simulink model "CAVE_MachE_Simulink_250904"  (R2024a)
settings: configuration reference "ConfigSetDesktopFixedStep" (kept outside this file)
PreLoadFcn:
  | VSS_BICYCLE=Simulink.Variant('Dual=0');
  | VSS_DUAL=Simulink.Variant('Dual=1');
  | Dual=1;
  | load('DriveCycle2.mat')
PostLoadFcn:
  | if any(exist('dsrtsu_mdlpostloadfcn', 'file') ~= 0), dsrtsu_mdlpostloadfcn('Execute', bdroot); end
InitFcn:
  | , if any(exist('rtifpga_mdlclblib', 'file') ~= 0), rtifpga_mdlclblib('Init', bdroot); end,
  | , if any(exist('dsmpb_private', 'file') ~= 0), dsmpb_private('dsmpb_mdlclblib', 'Init', bdroot); end,
  | load('DriveCycle2.mat')
model workspace (MAT data in the model file):
  Gas = 0.383333333333
undefined symbols (not defined in the file or in its folder): AccelCmd, ActTqLF_Nm_, ActTqLR_Nm_, ActTqRF_Nm_, ActTqRR_Nm_, BattChargeLimitMaxPwr, BattChargeLimitSocBpts, BattChargeLimitTbl, BattChrgCapcty, BattDischargeLimitSocBpts, BattDischargeLimitTbl, BattDischargeMaxPwr, BattNumCellsParallel, BattNumCellsSeries, BattOpenVoltCapBpts, BattOpenVoltTbl, BattResistSocBpts, BattResistTbl, BattResistTempBpts, BrakeMaxPrs, BrakeMaxTrq, ChassisDistCg2FrontAxle, ChassisDistCg2RearAxle, ChassisVehMass, CltchCmd, CoastDown, DecelCmd, DiffRatio, DiscIntNeverNeededParam, EnvGravCnst, EnvPrs, EnvTemp, FuelSpecificGrav, GearCmd, h, InitStates, lgSw, limitedMCT, MCT, MtrEffSpdBpts, MtrEffTbl, MtrEffTrqBpts, MtrPwrMax, MtrTrqMax, pMCT, RealSimPara, Ref_speed, Ref_time, SteeringCmd, SupvsryCtrlRegenBrkCutOffTbl, SupvsryCtrlRegenSpdBpts, TestScnrioCycleNum, US06, VEH
libraries: VSIGenLib x179, simulink x166, etargetslib x112, dsmpblib x58, vehdynlibtire x36, autolibshared x29, vehdynlibsuspension x21, vehdynlibtirecommon x21, autolibutils x15, CarMaker4SL x12, VsrLibWheel x12, autolibpowerinfoutils x9
(part 1 of 43)
PreSaveFcn:
  | , if any(exist('dsmpb_private', 'file') ~= 0), dsmpb_private('dsmpb_mdlclblib', 'PreSave', bdroot); end,
CloseFcn:
  | , if any(exist('dsmpb_private', 'file') ~= 0), dsmpb_private('dsmpb_mdlclblib', 'Close', bdroot); end,
settings Model: DataDictionary=DdPassengerEv.sldd  DSMPB_ID_DATA={'18088',struct('BlockId','f88c42c2-e70e-4436-bd85-ff34452e836e','SignalIds',{{'1df572a0-f117-4729-9091-2c1a0a26ec90','0824b86c-995c-4624-95de-4f5a118cf0f7','1af539eb-325a-4e38-9107-84d6b0267392','ebb0fa34-559f-4fe0-b409-8a817ae8753c','d7145080-d35d-4c02-8c9e-cf76ffb14dc2','5075bfde-4142-4aeb-b309-025b37120541','abbab0bd-1456-4252-a37b-ee5f55ea0579','b5d617b8-bb24-4539-9145-e591a0a295f8','7df03788-1936-4801-98c0-dd7f6dfcacba','19949bfb-f246-4995-90e8-29a3751a0fa7','9454b59a-aedd-4270-89a6-1cca43305823','37cf720c-23c2-4b6d-8589-7b035c806643','98db9f76-eafd-4d54-90d2-d997d73b87d4','ff589fc8-5b21-4798-a75e-d26fc35c1fa1','e61b2882-e27e-4f06-b730-5e5281621b34','6605e0e6-8bf3-4a45-a0b0-4b9c1cf463f3','0d0f5161-daad-47a1-bb1d-ec2adbc183ca','48ba6675-0966-4a1c-b127-4f76dca3de94','3c897f11-b2eb-4eb8-b88f-7b7e913c6e41','378f468e-364f-43c5-91f9-fc8ddef6aca6','9c7f20ac-956d-4c19-bdea-31a2a3930ea2','bc252920-9c7c-4b91-a017-ee1d69e3f03c','a5e7a104-8664-4690-a58a-7cbf05737866','fe1cfa34-9b23-4225-85e3-0403f07d36e7','ab40d80a-815e-4994-aacd-e42d283f5b3a','2a4143b2-c438-4d42-997d-0587141eb8f0','2686c37a-8724-40b3-99fb-f8873ba286b8','3707aa1b-88c1-4f14-8f25-f346aa75c252','7413af4b-f834-4020-ad34-3dd98c546e0c','3445835b-9a90-4408-a32d-d76b66b0385b','23c9a144-1259-4fa3-9a16-4a32a7eadff9','5b4206b0-ea89-4111-86f7-7a4fd8c76b72','85c84ea6-72b6-4ccb-9199-727b305580c3','97bb0073-9d03-44a9-972d-49a0eb465678','8c3f0698-b0b6-4624-aa00-3a3096f7cc2f','c968922f-253e-433f-ad46-daf21e902962','21ad150a-19dc-415b-bc1b-b39528ec9221','a3572415-9467-4ff8-a492-c6c1b3cb1b64','700ac678-fb53-40b6-8e97-9eeffe7a1ca8','14ed5f8b-aa1d-402b-b493-5622a729893d','bdbcc0b3-c6a4-485e-8fbf-8c12a8df89e7','7a19cc2b-f06b-466f-ae52-fb8ac6fb0258','87deda6a-2251-4462-8ae0-a20845c776d4','41874d9b-304a-4265-a3a1-69d5c58383ea'}}),'18719',struct('BlockId','79daabbd-4df4-4017-ba65-d977f7e6cd2f','SignalIds',{{'63c99320-3a8a-469e-8a50-5c577229603f'}}),'18720',struct('BlockId','9f21d727-31d5-41b9-aed1-27a40d8edf8b','SignalIds',{{'abab19c9-0d91-46eb-acba-2a4710e305d8'}}),'18721',struct('BlockId','5513e588-accc-447f-8233-209349c29c53','SignalIds',{{'cf7c35a9-6bda-4f5f-bfb5-f51ad44c376b'}}),'18722',struct('BlockId','a427ee23-ff95-4a9c-807f-ad2b61c33ee4','SignalIds',{{'b3e368f1-9670-4dd7-aa42-1fcccca64ddf'}}),'18723',struct('BlockId','53805a71-03ad-4b45-a2ab-66e4ec3700d0','SignalIds',{{'0801da20-d997-46db-8512-e37e1180e77c','d193450d-1a5a-4c8d-a2ac-d5fd306fefe3'}}),'18724',struct('BlockId','4d4909f9-4869-4ae2-8541-060fc5e29366','SignalIds',{{'0588d1ac-5d02-4ce0-9f56-5f4e572c1088','c0609b3e-104e-46bb-beb6-dc1d54d218ce','a0011887-c3f0-4769-95be-c916ccb77447','feb7a80d-e7d1-407d-8b44-49f086fb9d8a'}}),'42147',struct('BlockId','7c85148e-c3d7-432d-b81b-e11d436fb266','SignalIds',{{'d5c1f3b5-a22d-40e2-9adf-73dd3a0fe431'}}),'42148',struct('BlockId','5510fdf1-431a-410f-bcea-f7e8f570e2d1','SignalIds',{{'9fce7f97-eda7-4f24-878f-1a643d43b49c'}}),'42149',struct('BlockId','de0e2a2d-bbe1-43d1-85ae-8561a379e07c','SignalIds',{{'e73be657-c71a-4fa8-ab30-d8cdb28be71d'}}),'42224',struct('BlockId','1b1b092f-214b-4a80-b11b-37b75121e53b','SignalIds',{{'856b8b64-1382-4ba0-b818-e91eea7074c9'}}),'42225',struct('BlockId','cfba7721-c5cf-410b-a196-c40269978734','SignalIds',{{'7065876d-b123-4337-8b23-cec9822ec3f7'}}),'42226',struct('BlockId','45b8b98e-f988-42ef-b616-7180bc819cf2','SignalIds',{{'f4c7852e-b78f-4b21-ba9d-e4df57cf05c4'}}),'42232',struct('BlockId','ac7ecc60-8396-40a4-bc17-9f0f3c0759ca','SignalIds',{{'16a26856-ef2a-4966-8200-82aa3fe7ddbf'}}),'42233',struct('BlockId','13dab684-98bf-43e1-8dcd-5e4b904e530a','SignalIds',{{'2a6f66f1-336d-4450-a338-914a295f0636'}}),'42234',struct('BlockId','c2584fdd-8801-464b-b08c-93b745502641','SignalIds',{{'839033fa-96d7-490f-a336-e4074cb0a3a6'}}),'42263',struct('BlockId','5f5bdefb-1809-46da-bb29-06e43cb74cea','SignalIds',{{'9ba80473-de3d-4829-93f9-e3e4218e61ce'}}),'42264',struct('BlockId','3cf8559d-9792-4b7d-b1e9-07d3e8c975ef','SignalIds',{{'f258ffe4-6a36-4981-abe6-f58a11cec6e4'}}),'42772',struct('BlockId','2d079b89-a5d3-43f5-b2da-b67c6c9ddea6','SignalIds',{{'ca22f614-f5f3-4878-a32c-0e537783a285'}}),'42780',struct('BlockId','22a06564-7b80-437f-9a37-5f0480de49c5','SignalIds',{{'d3558271-70a3-4a15-b412-afa96387f019','02a3409b-9f87-437b-bf3a-cc29eabe585b','4dd1ea73-b952-4f27-91e5-448f679ccffd','2dcb7769-2bf3-4424-ac78-eb5f6dd54b66','045c974e-8d31-4d1e-8c69-be2d2594e84a'}}),'42781',struct('BlockId','f3d872af-dc59-442b-a387-2481dd52f459','SignalIds',{{'4ee2bd44-e8da-4e09-8a2d-8bab973be353','ce2328cf-0071-41cb-90b6-53c9d261887b'}}),'42785',struct('BlockId','b01cfdfa-14c4-45c6-876e-4dfb9db42377','SignalIds',{{'34ca8be0-54ab-4d71-8eb9-bde2ffc0f913'}}),'43275',struct('BlockId','53e01b05-b313-4d43-a0e9-b839859eb710','SignalIds',{{'161239c6-78c1-4aea-a8cb-c03beb6ae8ef'}}),'43351',struct('BlockId','937f730a-1a1f-4f40-8fb6-8c70050ca6d4','SignalIds',{{'ee16bc58-de2e-41bd-bfff-f1a6b1cd3b37','b53a6535-30cb-49b2-9826-525fa2ec09db','6c8ffc13-c120-49b6-9460-32fb34ba5a42','39b2e722-7db4-4c66-a473-01b75ecb1f7e','6185bd49-892f-4e96-a0db-104c5534c4be'}}),'53285',struct('BlockId','16d8a604-9c1c-446a-b099-d61de5aa33b6','SignalIds',{{'53a670ca-367a-4015-af59-0a4ccf6786c0'}}),'53286',struct('BlockId','0b674dd2-19ca-4446-b220-fc8d5b595023','SignalIds',{{'5b8c4e41-0d17-4777-94b0-82cdf3639591'}}),'53287',struct('BlockId','acc1cdc3-8447-4797-b99b-23f53584cd89','SignalIds',{{'798d274b-40e4-437a-8cff-3fe64b46bdee'}}),'53362',struct('BlockId','fa05054f-1d10-4053-a3ab-88de2181fb62','SignalIds',{{'62d7a703-6a80-4bb3-8c94-4aa286060642'}}),'53363',struct('BlockId','592b8698-2132-4534-b0cb-f397cafefe99','SignalIds',{{'7bf88a02-66e7-4ac9-b07b-8ef5c3f39ebe'}}),'53364',struct('BlockId','ed7f7bf4-c332-4eaf-b7a0-9a3e39ff220c','SignalIds',{{'14614c0f-4dcb-41ad-888f-44d9410ff755'}}),'53370',struct('BlockId','46b7a166-361a-4c63-987b-9c5458ecc9a1','SignalIds',{{'3b0f4705-2f11-47b6-a9d5-53db34d59c31'}}),'53371',struct('BlockId','ae3904f3-e5f6-4d76-ade0-dc026faaa291','SignalIds',{{'7e24304b-b1e8-45eb-8b0c-af013d2d4bda'}}),'53372',struct('BlockId','c54e3026-0271-4358-9411-7041e7617221','SignalIds',{{'5e86e281-beb7-4af3-8f70-5c64a7b53fca'}}),'53401',struct('BlockId','2b06d236-438c-47d1-a5ed-a3b4029e53ea','SignalIds',{{'a5e319cf-b6c5-4820-9d47-2095d71b5beb'}}),'53402',struct('BlockId','13fd95eb-2a12-44a2-a228-d32be911dec2','SignalIds',{{'1e51e76a-d542-4893-acc0-271136175a32'}}),'53938',struct('BlockId','b9601c81-6b9a-4899-9674-d210556d02fb','SignalIds',{{'0558f8c2-4cca-4e5f-b993-2218a1539cc0'}}),'53946',struct('BlockId','f48ff196-73d7-4a07-92f5-53213a8a1e9b','SignalIds',{{'e624b599-2a19-43d1-a641-6652fb717343','86c8dfcf-8be1-4b0d-a2d0-371f42dc5516','b3dbc52b-6c0c-4cc6-a444-a29ece183bd9','43f629a9-07fd-4073-8fcd-45d3ce21c3b6','5e19b6f7-3038-45c6-8e3e-ef045c05b4fd'}}),'53947',struct('BlockId','6c938526-259f-41e9-a2f8-a14abf91ee50','SignalIds',{{'b0c46e42-55c2-4d88-9152-52659a562abf','5b5d6a18-e6c9-42c2-9788-ac69392afa6a'}}),'53951',struct('BlockId','08b86b6e-296e-4239-8997-a10b8d0ddd08','SignalIds',{{'4ae611ee-6197-41a3-9d31-87a04b9315f1'}}),'54441',struct('BlockId','b04af7f2-b95e-4b9b-b864-675cbd35c9b4','SignalIds',{{'bde72e54-00c5-4010-b7ca-ff93c988600a'}}),'54517',struct('BlockId','122e4405-43be-4c96-9c54-eb8ae7ed9e1b','SignalIds',{{'9766567d-d17c-4cf7-8a96-377d27c1abc9','d557bff4-8d9a-479f-8743-9915a9fdcfcb','355d3337-bde6-407c-98b2-719146037029','9d880830-ba4d-420a-9aea-edc847cdc4a2','60a580ab-cf97-4422-bb0e-e9b315a713d1'}}),'56968',struct('BlockId','d99e0ded-f5a5-46a8-b396-92444fc34f63','SignalIds',{{'7aa56a6d-5ee3-458c-bef6-5989bf324280'}}),'56969',struct('BlockId','60f64cb9-aea7-4596-af31-dc9d1caa6371','SignalIds',{{'7b34ff50-2b4a-413a-84bd-262a19c54096'}}),'56970',struct('BlockId','d09ab556-90e0-425e-8b97-314c2acf9fd6','SignalIds',{{'35ba5fe2-8c28-414e-bb09-024425fbca9a'}}),'57045',struct('BlockId','3988e426-b89f-4555-a48c-4c7e4846a701','SignalIds',{{'4474300f-5e28-4694-8e90-a56782fffb09'}}),'57046',struct('BlockId','169b0f1a-8b92-4a60-a4b9-86b0e8e2e508','SignalIds',{{'819d2bde-2325-45a7-adaf-9b54c1085683'}}),'57047',struct('BlockId','f5ba7f68-e0e8-444e-baff-31376305e226','SignalIds',{{'ba4ec118-1415-4332-b360-58e54faaec65'}}),'57053',struct('BlockId','3bcd854f-b759-4de1-a69c-aca1010de7b2','SignalIds',{{'30163c60-9aba-4782-8ac4-d3a993b94bdc'}}),'57054',struct('BlockId','7c36409e-4522-4cd0-b3e4-e035f492daf8','SignalIds',{{'f2504b65-ea43-4bb3-985e-e6e603cb8553'}}),'57055',struct('BlockId','0c5a6c3a-07a7-465c-b30d-22d6b5400665','SignalIds',{{'432be6db-6dd4-45fc-88f5-a3e0ec4dc183'}}),'57084',struct('BlockId','11524a80-2d22-430c-88a5-77d1a826bee5','SignalIds',{{'9618a70e-79e2-467a-9325-3bbceee6012a'}}),'57085',struct('BlockId','a4ee9257-809b-4fe0-89fd-f39f8e736e3d','SignalIds',{{'8f19cee1-6754-4d3e-b015-3e015bd096d0'}}),'57621',struct('BlockId','db91067d-8c34-4fb2-85fc-271bfb3ef537','SignalIds',{{'68315c7b-de4f-4653-abbc-388c29f7989f'}}),'57629',struct('BlockId','b9a2d293-7261-4aa5-ba50-7ae3a2ab8763','SignalIds',{{'04b2a66a-a532-43ae-88c1-48baac6dbd03','8b2ff3d3-0f4a-4b50-ac95-e18a93028560','6a35b15d-d20d-42cb-87fd-945b2d231bb3','2530bbe1-d2ca-4b1f-833d-7c33051135d3','9724ba46-53b5-40e8-bc04-f7d92899bd8a'}}),'57630',struct('BlockId','0b6ecde8-1e1b-44b1-8439-454900b059b9','SignalIds',{{'898e4ed5-2f18-4226-b222-a500e6649cd2','575bae4b-fc0f-4f35-a9eb-1be285fa7764'}}),'57634',struct('BlockId','148464f6-7764-48b9-989f-a4e13b114287','SignalIds',{{'193b56cd-482a-4c57-8534-7daca0748b44'}}),'58124',struct('BlockId','4871e5c1-70b1-4ce4-8de1-993df5081cd9','SignalIds',{{'699433aa-efe8-464b-a9fd-08b20d29c9da'}}),'58200',struct('BlockId','62509075-e4e8-4f7a-97c0-d58bf19eae4f','SignalIds',{{'ea0eab5e-7952-4dfe-9d9e-42987e4c006a','f61d5f86-e912-4fa6-b053-78fbd65945af','7d1181af-344b-4887-be45-fdc8e0e6f4d6','82dcb495-664a-43d6-9d56-bdca6e579333','50d72421-119a-428f-a4ad-1d9dd8a9a7c4'}})}  RTICANMMDATA=struct('GeneralSetupData',struct('modelroot','C:\GitDev\Anye\cave_carla_dev\Vehicles\VehicleProjects\Bolt_EV\System','generalsettings',struct('filesettings',struct('destfolder',struct('Name','RTICANMM_FILES','Check',1),'buildfolder',struct('Name','.','Check',1),'AbsDestfolder',struct('Name','C:\GitDev\Anye\cave_carla_dev\Vehicles\VehicleProjects\Bolt_EV\System\RTICANMM_FILES'),'AbsBuildfolder',struct('Name','C:\GitDev\Anye\cave_carla_dev\Vehicles\VehicleProjects\Bolt_EV\System'))),'options',struct('addpaths',1,'rmpaths',1,'addtrcexclusion',true,'cannavigator',struct('checkmonitoring',0),'show_usrtrc',0,'use_usrtrc',0),'advanced',struct('options',ones(1,100)),'MPSetup',{{}},'RTI',struct('Type','DSRT','Ver','4.2p1','Date','11-Feb-2020'),'modelname','CAVE_MachE','block','CAVE_MachE'))  DSRTSU_INTERNAL_RTIFPGA=210  DSRTSU_INTERNAL_RTISTBM_VER=24.1  PauseTimes=45  Creator=9bt  LastModifiedBy=yusun
settings ConfigSetRef: SourceName=ConfigSetDesktopFixedStep

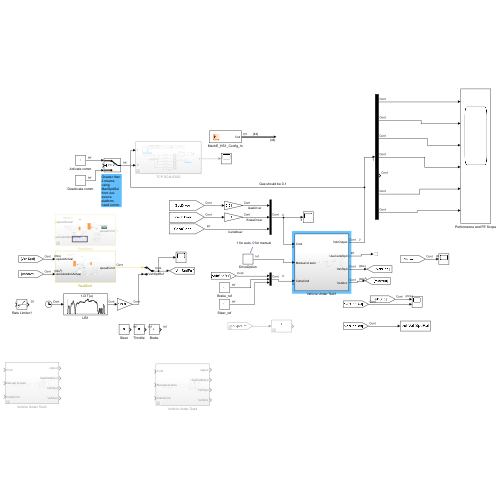
[thumbnail: Simulink's stored preview of the top-level diagram]
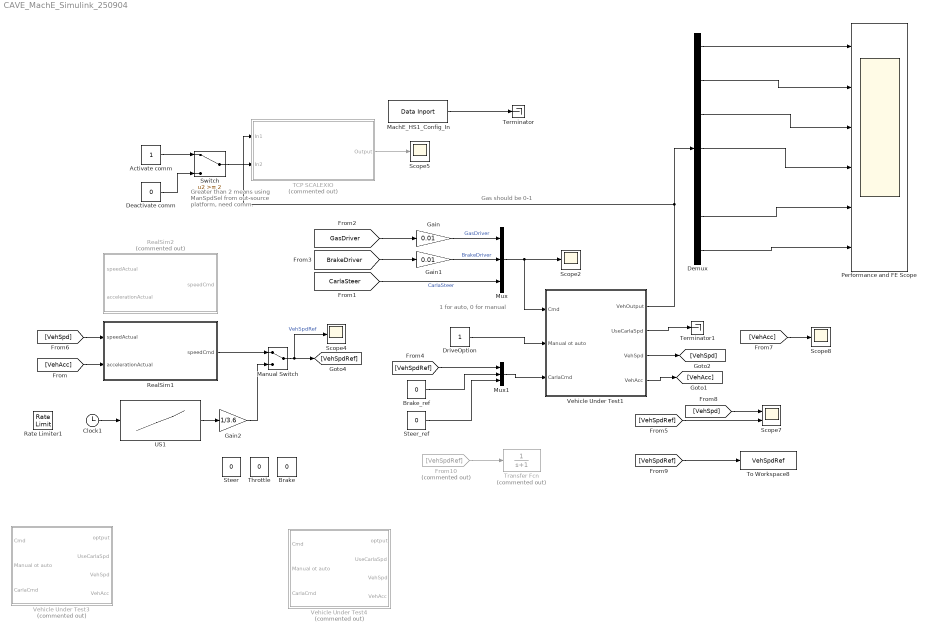
== system CAVE_MachE_Simulink_250904 ==
  note: Greater than 2 means using ManSpdSel from out-source platform, need comm.
  note: 1 for auto, 0 for manual
  note: Gas should be 0-1
  Activate comm : Constant
  Brake : Constant  Value=0
  Brake_ref : Constant  Value=0
  Clock1 : Clock
  Deactivate comm : Constant  Value=0
  Demux : Demux  Outputs=7
  DriveOption : Constant
  From10 : From  Commented=on  GotoTag=VehSpdRef
  Gain : Gain  Gain=0.01
  Gain1 : Gain  Gain=0.01
  Gain2 : Gain  Gain=1/3.6
  MachE_HS1_Config_In : dsmpblib/Data Inport  Priority=10000
      settings: SourceProductName=dSPACE Model Interface Package for Simulink (MIPS)
  Manual Switch : ManualSwitch
  Mux : Mux  Inputs=3
  Mux1 : Mux  Inputs=3
  Performance and FE Scope : Scope  NumInputPorts=6
  Rate Limiter1 : RateLimiter  RisingSlewLimit=4  FallingSlewLimit=-4  SampleTimeMode=inherited
  RealSim1 : Subsystem
  RealSim2 : Subsystem  Commented=on
  Scope{2,4..5,8} (4 alike) : Scope
  Scope7 : Scope  NumInputPorts=2
  Steer : Constant  Value=0
  Steer_ref : Constant  Value=0
  Switch : Switch  Threshold=2  SaturateOnIntegerOverflow=off  InputSameDT=off
  TCP SCALEXIO : Subsystem  Commented=on
  Terminator : Terminator
  Terminator1 : Terminator
  Throttle : Constant  Value=0
  To Workspace8 : ToWorkspace  VariableName=VehSpdRef  SaveFormat=Timeseries  SampleTime=0.1
  Transfer Fcn : TransferFcn  Commented=on  Denominator=[1 1]
  US1 : Lookup_n-D  NumberOfTableDimensions=1  BreakpointsForDimension1=US06.Time  Table=US06.Speed  InternalRulePriority=Speed  RndMeth=Simplest
  Vehicle Under Test1 : Subsystem
  Vehicle Under Test3 : Subsystem  Commented=on
  Vehicle Under Test4 : Subsystem  Commented=on
  wires:
  Mux/1 -> Vehicle Under Test1/1(Cmd), Scope2/1
  DriveOption/1 -> Vehicle Under Test1/2(Manual ot auto)
  [GasDriver] -> Gain/1
  [BrakeDriver] -> Gain1/1
  MachE_HS1_Config_In/1 -> Terminator/1
  Gain/1 -> Mux/1  "GasDriver"
  Gain1/1 -> Mux/2  "BrakeDriver"
  Vehicle Under Test1/1(VehOutput) -> TCP SCALEXIO/1(In1), Demux/1
  Switch/1 -> TCP SCALEXIO/2(In2)
  TCP SCALEXIO/1(Output) -> Scope5/1
  Deactivate comm/1 -> Switch/3
  Activate comm/1 -> Switch/1
  [CarlaSteer] -> Mux/3  "CarlaSteer"
  Manual Switch/1 -> Scope4/1, [VehSpdRef]  "VehSpdRef"
  US1/1 -> Gain2/1
  RealSim1/1(speedCmd) -> Manual Switch/1
  [VehAcc] -> RealSim1/2(accelerationActual)
  [VehSpd] -> RealSim1/1(speedActual)
  [VehSpdRef] -> Mux1/1
  Mux1/1 -> Vehicle Under Test1/3(CarlaCmd)
  Vehicle Under Test1/4(VehAcc) -> [VehAcc]
  Steer_ref/1 -> Mux1/3
  Brake_ref/1 -> Mux1/2
  Vehicle Under Test1/2(UseCarlaSpd) -> Terminator1/1
  Clock1/1 -> US1/1
  [VehSpdRef] -> Scope7/2
  Gain2/1 -> Manual Switch/2
  Demux/1 -> Performance and FE Scope/1
  Demux/7 -> Performance and FE Scope/6
  Demux/6 -> Performance and FE Scope/5
  Demux/4 -> Performance and FE Scope/4
  Demux/3 -> Performance and FE Scope/3
  Demux/2 -> Performance and FE Scope/2
  [VehAcc] -> Scope8/1
  [VehSpd] -> Scope7/1
  [VehSpdRef] -> To Workspace8/1
  From10/1 -> Transfer Fcn/1
  Vehicle Under Test1/3(VehSpd) -> [VehSpd]

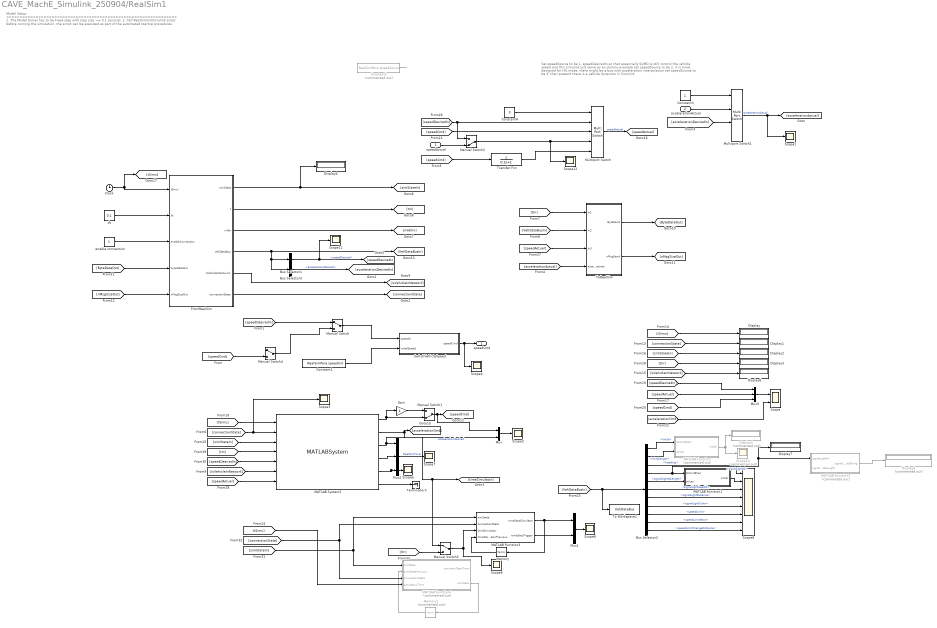
== system CAVE_MachE_Simulink_250904/RealSim1 ==
  note: Set speedSource to be 1, speedDesiredIn so that essentially SUMO is still control the vehicle speed and this simulink just serve as an dummy example
      |
      | set speedSource to be 2, it is more designed for HIL mode, there might be a bug with acceleration interpolation
      |
      | set speedSource to be 3, then pretend there is a vehicle dynamics in Simulink
  note: Model Setup
      | ================================================================
      | 1. The Model Solver has to be Fixed-step with step size <= 0.1 seconds.
      | 2. Call RealSimInitSimulink script before running the simulation. the script can be executed as part of the automated startup procedures.
  speedActual : Inport
  accelerationActual : Inport  Port=2
  Bus Selector1 : BusSelector  OutputSignals=speedDesired
  Bus Selector2 : BusSelector  OutputSignals=linkId,linkIdLength,heading,signalLightId,signalLightIdLength,signalLightHeadId,signalLightDistance,signalLightColor,speedLimit,speedLimitNext,speedLimitChangeDistance
  Bus Selector3 : BusSelector  OutputSignals=accelerationDesired
  Clock : Clock
  Constant1 : Constant  Value=RealSimPara.speedInit
  Constant2 : Constant  Commented=on  Value=RealSimPara.speedSource
  Constant3 : Constant
  Constant4 : Constant  Value=3
  Display{,1..4,6..7} (7 alike) : Display
  Display5 : Display  Commented=on
  Display9 : Display  Commented=on
  FromRealSim : Subsystem
  Gain : Gain
  MATLAB Function : MATLAB Function  Commented=on  TreatAsAtomicUnit=on
  MATLAB Function1 : MATLAB Function  TreatAsAtomicUnit=on
  MATLAB Function2 : MATLAB Function  Commented=on  TreatAsAtomicUnit=on  SystemSampleTime=0.001
  MATLAB Function3 : MATLAB Function  TreatAsAtomicUnit=on
  MATLAB Function4 : MATLAB Function  Commented=on  TreatAsAtomicUnit=on
  MATLAB System2 : MATLABSystem  System=RealSimInterpSpeed  initialSpeed=RealSimPara.speedInit  speedLookAheadHorizon=RealSimPara.tLookahead  speedUpperBound=30  smoothWindow=RealSimPara.smoothWindow  SimulateUsing=Interpreted execution
      mask Type: RealSimInterpSpeed
      mask Display:
      | disp('RealSimInterpSpeed');
      | port_label('input',1,'simulationTime');
      | port_label('input',2,'connectionState');
      | port_label('input',3,'simState');
      | port_label('input',4,'timeReceive');
      | port_label('input',5,'speedReceive');
      | port_label('input',6,'isVehicleInNetwork');
      | port_label('input',7,'speedActual');
      | port_label('output',1,'speedLookAhead');
      | port_label('output',2,'accelerationDesired');
      | port_label('output',3,'timeSimulator');
      | port_label('output',4,'timeStepSimulator');
      | port_label('output',5,'timeStepTrigger');
      | port_label('output',6,'RealSimDelay');
  Manual Switch : ManualSwitch
  Manual Switch1 : ManualSwitch  CurrentSetting=0
  Manual Switch2 : ManualSwitch  CurrentSetting=0
  Manual Switch3 : ManualSwitch
  Manual Switch4 : ManualSwitch
  Memory : Memory
  Memory1 : Memory  Commented=on
  Multiport Switch : MultiPortSwitch  Inputs=4  SaturateOnIntegerOverflow=off  InputSameDT=off
  Multiport Switch1 : MultiPortSwitch  SaturateOnIntegerOverflow=off  InputSameDT=off
  Mux : Mux  Inputs=2
  Mux1 : Mux  Inputs=2
  Mux2 : Mux  Inputs=3
  Mux3 : Mux  Inputs=3
  Scope : Scope  NumInputPorts=2
  Scope{1..7,9,11..12} (10 alike) : Scope
  Scope10 : Scope  Commented=on
  Scope8 : Scope  NumInputPorts=8
  SwitchVehicleSpeed : Subsystem
  Terminator3 : Terminator
  To Workspace1 : ToWorkspace  VariableName=VehDataBus  SaveFormat=Timeseries  SampleTime=-1
  ToRealSim : Subsystem
  Transfer Fcn : TransferFcn  Denominator=[0.1 1]
  dt : Constant  Value=0.1
  enable connection : Constant
  speedCmd : Outport
  wires:
  [speedCmd] -> Manual Switch4/2
  Manual Switch3/1 -> MATLAB Function3/3(timeSimulator), Scope9/1
  [tIn] -> Manual Switch3/2
  MATLAB Function4/2(simState) -> Memory1/1
  Memory1/1 -> MATLAB Function4/2(simStatePrevious)
  MATLAB Function3/2(timeStepTrigger) -> Mux1/2
  Mux1/1 -> Scope6/1
  Memory/1 -> MATLAB Function3/4(timeStepSimulatorPrevious)
  MATLAB Function3/1(timeStepSimulator) -> Memory/1, Mux1/1
  [simStateIn] -> MATLAB Function3/1(simState), MATLAB Function4/1("simState ")
  [connectionState] -> MATLAB Function3/2(connectionState), MATLAB Function4/3(connectionState)
  [tSimu] -> MATLAB Function4/4(simulationTime)
  Transfer Fcn/1 -> Multiport Switch/5
  [speedCmd] -> Transfer Fcn/1
  speedActual/1 -> Manual Switch2/2
  Mux/1 -> Scope2/1
  FromRealSim/6(connectionState) -> [connectionState]
  Multiport Switch1/1 -> [accelerationActual], Scope1/1  "accelerationActual"
  accelerationActual/1 -> Multiport Switch1/2
  [accelerationDesiredIn] -> Multiport Switch1/3
  Constant3/1 -> Multiport Switch1/1
  Bus Selector3/1 -> [accelerationDesiredIn]  "<accelerationDesired>"
  Manual Switch/1 -> SwitchVehicleSpeed/1(speedIn)
  SwitchVehicleSpeed/1(speedCmd) -> speedCmd/1, Scope4/1
  Constant1/1 -> SwitchVehicleSpeed/2(initialSpeed)
  [speedDesiredIn] -> Manual Switch/1
  Manual Switch4/1 -> Manual Switch/2
  Constant2/1 -> ?
  ? -> MATLAB Function2/2(signalLightIdLength)
  [simStateIn] -> Display2/1
  Mux3/1 -> Scope/1
  [isVehicleInNetwork] -> MATLAB System2/6
  Bus Selector2/3 -> Scope8/1  "<heading>"
  MATLAB Function1/1(intVal) -> Scope8/2
  ToRealSim/1(ByteSend) -> [ByteDataOut]
  [accelerationActual] -> ToRealSim/4(accelerationDesired)
  Bus Selector2/6 -> Scope8/3  "<signalLightHeadId>"
  Multiport Switch/1 -> [speedActual]  "speedActual"
  [VehDataBusIn] -> ToRealSim/2(In2)
  [accelerationCmd] -> Scope/2
  FromRealSim/5(isVehicleInNetwork) -> [isVehicleInNetwork]
  FromRealSim/2(t) -> [tIn]
  [speedActual] -> ToRealSim/3(In3)
  FromRealSim/1(simState) -> [simStateIn], Display4/1
  ToRealSim/2(nMsgSend) -> [nMsgSizeOut]
  Manual Switch1/1 -> [speedCmd], Mux/1
  Constant4/1 -> Multiport Switch/1
  [speedCmd] -> Mux3/3
  [tIn] -> MATLAB System2/4
  Bus Selector2/2 -> MATLAB Function/2(strLen)  "<linkIdLength>"
  MATLAB Function2/1(signalLightIdString) -> Display9/1
  MATLAB System2/2 -> Mux/2, [accelerationCmd]  "accelerationDesired"
  [tIn] -> ToRealSim/1(In1)
  Bus Selector2/1 -> MATLAB Function/1(strUint8Vec)  "<linkId>"
  MATLAB System2/6 -> Terminator3/1
  [connectionState] -> Scope3/1, MATLAB System2/2
  Manual Switch2/1 -> Multiport Switch/4, Scope12/1
  Bus Selector2/8 -> Scope8/5  "<signalLightColor>"
  MATLAB System2/4 -> Mux2/2
  Bus Selector2/7 -> Scope8/4  "<signalLightDistance>"
  [tIn] -> Display3/1
  Clock/1 -> [tSimu], FromRealSim/1(tSimu)
  [connectionState] -> Display1/1
  [speedActual] -> Mux3/2
  FromRealSim/3(nVeh) -> [nVehIn]
  [speedActual] -> MATLAB System2/7
  [speedDesiredIn] -> Multiport Switch/2, Manual Switch2/1
  Bus Selector2/11 -> Scope8/8  "<speedLimitChangeDistance>"
  [nMsgSizeOut] -> FromRealSim/5(nMsgSizeOut)
  [speedDesiredIn] -> MATLAB System2/5
  MATLAB Function/1(intVal) -> Display5/1, Scope10/1
  enable connection/1 -> FromRealSim/3(enableConnection)
  FromRealSim/4(VehDataBus) -> Bus Selector3/1, Bus Selector1/1, [VehDataBusIn]
  Bus Selector2/10 -> Scope8/7  "<speedLimitNext>"
  dt/1 -> FromRealSim/2(dt)
  MATLAB System2/3 -> Mux2/1, Manual Switch3/1, [timeSimulator]
  Bus Selector2/4 -> MATLAB Function1/1(strUint8Vec), MATLAB Function2/1(signalLightId), Display7/1  "<signalLightId>"
  [speedDesiredIn] -> Mux3/1
  Bus Selector2/9 -> Scope8/6  "<speedLimit>"
  Bus Selector1/1 -> [speedDesiredIn], Scope11/1  "<speedDesired>"
  Gain/1 -> Manual Switch1/1
  [tSimu] -> MATLAB System2/1
  Mux2/1 -> Scope7/1  "RealSimTime"
  [speedCmd] -> Multiport Switch/3
  MATLAB System2/1 -> Manual Switch1/2, Gain/1
  [VehDataBusIn] -> Bus Selector2/1, To Workspace1/1
  MATLAB System2/5 -> Mux2/3, Scope5/1
  [ByteDataOut] -> FromRealSim/4(byteDataOut)
  [isVehicleInNetwork] -> Display6/1
  [simStateIn] -> MATLAB System2/3
  Bus Selector2/5 -> MATLAB Function1/2(strLen)  "<signalLightIdLength>"
  [tSimu] -> Display/1

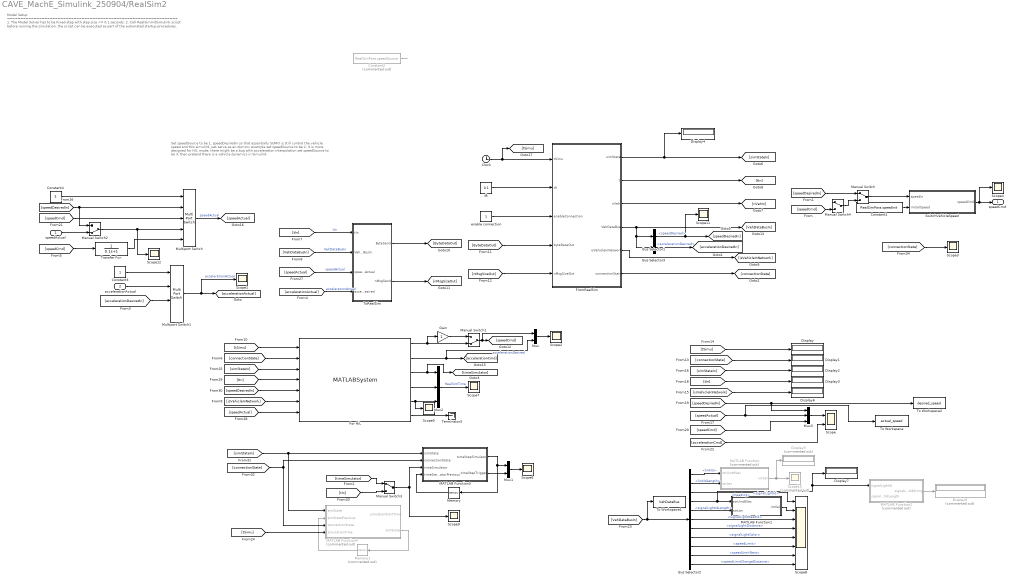
== system CAVE_MachE_Simulink_250904/RealSim2 ==
  note: Set speedSource to be 1, speedDesiredIn so that essentially SUMO is still control the vehicle speed and this simulink just serve as an dummy example
      |
      | set speedSource to be 2, it is more designed for HIL mode, there might be a bug with acceleration interpolation
      |
      | set speedSource to be 3, then pretend there is a vehicle dynamics in Simulink
  note: Model Setup
      | ================================================================
      | 1. The Model Solver has to be Fixed-step with step size <= 0.1 seconds.
      | 2. Call RealSimInitSimulink script before running the simulation. the script can be executed as part of the automated startup procedures.
  speedActual : Inport
  accelerationActual : Inport  Port=2
  Bus Selector1 : BusSelector  OutputSignals=speedDesired
  Bus Selector2 : BusSelector  OutputSignals=linkId,linkIdLength,heading,signalLightId,signalLightIdLength,signalLightHeadId,signalLightDistance,signalLightColor,speedLimit,speedLimitNext,speedLimitChangeDistance
  Bus Selector3 : BusSelector  OutputSignals=accelerationDesired
  Clock : Clock
  Constant1 : Constant  Value=RealSimPara.speedInit
  Constant2 : Constant  Commented=on  Value=RealSimPara.speedSource
  Constant3 : Constant
  Constant4 : Constant  Value=3
  Display{,1..4,6..7} (7 alike) : Display
  Display5 : Display  Commented=on
  Display9 : Display  Commented=on
  For HiL : MATLABSystem  System=RealSimInterpSpeed  initialSpeed=RealSimPara.speedInit  speedLookAheadHorizon=RealSimPara.tLookahead  speedUpperBound=30  smoothWindow=RealSimPara.smoothWindow  SimulateUsing=Interpreted execution
      mask Type: RealSimInterpSpeed
      mask Display:
      | disp('RealSimInterpSpeed');
      | port_label('input',1,'simulationTime');
      | port_label('input',2,'connectionState');
      | port_label('input',3,'simState');
      | port_label('input',4,'timeReceive');
      | port_label('input',5,'speedReceive');
      | port_label('input',6,'isVehicleInNetwork');
      | port_label('input',7,'speedActual');
      | port_label('output',1,'speedLookAhead');
      | port_label('output',2,'accelerationDesired');
      | port_label('output',3,'timeSimulator');
      | port_label('output',4,'timeStepSimulator');
      | port_label('output',5,'timeStepTrigger');
      | port_label('output',6,'RealSimDelay');
  FromRealSim : Subsystem
  Gain : Gain
  MATLAB Function : MATLAB Function  Commented=on  TreatAsAtomicUnit=on
  MATLAB Function1 : MATLAB Function  TreatAsAtomicUnit=on
  MATLAB Function2 : MATLAB Function  Commented=on  TreatAsAtomicUnit=on  SystemSampleTime=0.001
  MATLAB Function3 : MATLAB Function  TreatAsAtomicUnit=on
  MATLAB Function4 : MATLAB Function  Commented=on  TreatAsAtomicUnit=on
  Manual Switch : ManualSwitch
  Manual Switch1 : ManualSwitch  CurrentSetting=0
  Manual Switch2 : ManualSwitch  CurrentSetting=0
  Manual Switch3 : ManualSwitch
  Manual Switch4 : ManualSwitch
  Memory : Memory
  Memory1 : Memory  Commented=on
  Multiport Switch : MultiPortSwitch  Inputs=4  SaturateOnIntegerOverflow=off  InputSameDT=off
  Multiport Switch1 : MultiPortSwitch  SaturateOnIntegerOverflow=off  InputSameDT=off
  Mux : Mux  Inputs=2
  Mux1 : Mux  Inputs=2
  Mux2 : Mux  Inputs=3
  Mux3 : Mux  Inputs=3
  Scope : Scope  NumInputPorts=2
  Scope{1..7,9,11..12} (10 alike) : Scope
  Scope10 : Scope  Commented=on
  Scope8 : Scope  NumInputPorts=8
  SwitchVehicleSpeed : Subsystem
  Terminator3 : Terminator
  To Workspace : ToWorkspace  VariableName=actual_speed  SaveFormat=Timeseries  SampleTime=0.1
  To Workspace1 : ToWorkspace  VariableName=VehDataBus  SaveFormat=Timeseries  SampleTime=-1
  To Workspace2 : ToWorkspace  VariableName=desired_speed  SaveFormat=Timeseries  SampleTime=0.1
  ToRealSim : Subsystem
  Transfer Fcn : TransferFcn  Denominator=[0.1 1]
  dt : Constant  Value=0.1
  enable connection : Constant
  speedCmd : Outport
  wires:
  [speedCmd] -> Manual Switch4/2
  Manual Switch3/1 -> MATLAB Function3/3(timeSimulator), Scope9/1
  [tIn] -> Manual Switch3/2
  MATLAB Function4/2(simState) -> Memory1/1
  Memory1/1 -> MATLAB Function4/2(simStatePrevious)
  MATLAB Function3/2(timeStepTrigger) -> Mux1/2
  Mux1/1 -> Scope6/1
  Memory/1 -> MATLAB Function3/4(timeStepSimulatorPrevious)
  MATLAB Function3/1(timeStepSimulator) -> Memory/1, Mux1/1
  [simStateIn] -> MATLAB Function4/1("simState "), MATLAB Function3/1(simState)
  [connectionState] -> MATLAB Function3/2(connectionState), MATLAB Function4/3(connectionState)
  [tSimu] -> MATLAB Function4/4(simulationTime)
  Transfer Fcn/1 -> Multiport Switch/5
  [speedCmd] -> Transfer Fcn/1
  speedActual/1 -> Manual Switch2/2
  Mux/1 -> Scope2/1
  FromRealSim/6(connectionState) -> [connectionState]
  Multiport Switch1/1 -> [accelerationActual], Scope1/1  "accelerationActual"
  accelerationActual/1 -> Multiport Switch1/2
  [accelerationDesiredIn] -> Multiport Switch1/3
  Constant3/1 -> Multiport Switch1/1
  Bus Selector3/1 -> [accelerationDesiredIn]  "<accelerationDesired>"
  Manual Switch/1 -> SwitchVehicleSpeed/1(speedIn)
  SwitchVehicleSpeed/1(speedCmd) -> speedCmd/1, Scope4/1
  Constant1/1 -> SwitchVehicleSpeed/2(initialSpeed)
  [speedDesiredIn] -> Manual Switch/1
  Manual Switch4/1 -> Manual Switch/2
  Constant2/1 -> ?
  [simStateIn] -> Display2/1
  Mux3/1 -> Scope/1
  [isVehicleInNetwork] -> For HiL/6
  Bus Selector2/3 -> Scope8/1  "<heading>"
  MATLAB Function1/1(intVal) -> Scope8/2
  ToRealSim/1(ByteSend) -> [ByteDataOut]
  [accelerationActual] -> ToRealSim/4(accelerationDesired)  "accelerationActual"
  Bus Selector2/6 -> Scope8/3  "<signalLightHeadId>"
  Multiport Switch/1 -> [speedActual]  "speedActual"
  [VehDataBusIn] -> ToRealSim/2(VehDataBusIn)  "VehDataBusIn"
  [accelerationCmd] -> Scope/2
  FromRealSim/5(isVehicleInNetwork) -> [isVehicleInNetwork]
  FromRealSim/2(t) -> [tIn]
  [speedActual] -> ToRealSim/3(speedActual)  "speedActual"
  FromRealSim/1(simState) -> [simStateIn], Display4/1
  ToRealSim/2(nMsgSend) -> [nMsgSizeOut]
  Manual Switch1/1 -> [speedCmd], Mux/1
  Constant4/1 -> Multiport Switch/1
  [speedCmd] -> Mux3/3
  [tIn] -> For HiL/4
  Bus Selector2/2 -> MATLAB Function/2(strLen)  "<linkIdLength>"
  MATLAB Function2/1(signalLightIdString) -> Display9/1
  For HiL/2 -> Mux/2, [accelerationCmd]  "accelerationDesired"
  [tIn] -> ToRealSim/1(tIn)  "tIn"
  Bus Selector2/1 -> MATLAB Function/1(strUint8Vec)  "<linkId>"
  For HiL/6 -> Terminator3/1
  [connectionState] -> For HiL/2
  Manual Switch2/1 -> Multiport Switch/4, Scope12/1
  Bus Selector2/8 -> Scope8/5  "<signalLightColor>"
  For HiL/4 -> Mux2/2
  Bus Selector2/7 -> Scope8/4  "<signalLightDistance>"
  [tIn] -> Display3/1
  Clock/1 -> [tSimu], FromRealSim/1(tSimu)
  [connectionState] -> Display1/1
  [speedActual] -> Mux3/2, To Workspace/1
  FromRealSim/3(nVeh) -> [nVehIn]
  [speedActual] -> For HiL/7
  [speedDesiredIn] -> Multiport Switch/2, Manual Switch2/1
  Bus Selector2/11 -> Scope8/8  "<speedLimitChangeDistance>"
  [nMsgSizeOut] -> FromRealSim/5(nMsgSizeOut)
  [speedDesiredIn] -> For HiL/5
  MATLAB Function/1(intVal) -> Scope10/1, Display5/1
  enable connection/1 -> FromRealSim/3(enableConnection)
  FromRealSim/4(VehDataBus) -> [VehDataBusIn], Bus Selector1/1, Bus Selector3/1
  Bus Selector2/10 -> Scope8/7  "<speedLimitNext>"
  dt/1 -> FromRealSim/2(dt)
  For HiL/3 -> [timeSimulator], Mux2/1
  Bus Selector2/4 -> MATLAB Function1/1(strUint8Vec), MATLAB Function2/1(signalLightId), Display7/1  "<signalLightId>"
  [speedDesiredIn] -> Mux3/1, To Workspace2/1
  Bus Selector2/9 -> Scope8/6  "<speedLimit>"
  Bus Selector1/1 -> [speedDesiredIn], Scope11/1  "<speedDesired>"
  Gain/1 -> Manual Switch1/1
  [tSimu] -> For HiL/1
  Mux2/1 -> Scope7/1  "RealSimTime"
  [speedCmd] -> Multiport Switch/3
  For HiL/1 -> Gain/1, Manual Switch1/2
  [VehDataBusIn] -> To Workspace1/1, Bus Selector2/1
  For HiL/5 -> Mux2/3, Scope5/1
  [ByteDataOut] -> FromRealSim/4(byteDataOut)
  [isVehicleInNetwork] -> Display6/1
  [simStateIn] -> For HiL/3
  Bus Selector2/5 -> MATLAB Function1/2(strLen)  "<signalLightIdLength>"
  [tSimu] -> Display/1
  [timeSimulator] -> Manual Switch3/1
  [connectionState] -> Scope3/1

== system CAVE_MachE_Simulink_250904/TCP SCALEXIO ==
  note: Receiving gas, brake, steering; or three identical speeds
  note: Sending out x, y, heading, time, and speed
  In1 : Inport
  In2 : Inport  Port=2
  Constant2 : Constant  Value=zeros(1004,1);  OutDataTypeStr=uint8
  Data Type Conversion1 : DataTypeConversion  OutDataTypeStr=double  SaturateOnIntegerOverflow=off  RndMeth=Floor
  Data Type Conversion2 : DataTypeConversion  SaturateOnIntegerOverflow=off  RndMeth=Floor
  Data Type Conversion3 : DataTypeConversion  OutDataTypeStr=boolean  SaturateOnIntegerOverflow=off  RndMeth=Floor
  Defloater{,1..4} (5 alike) : VSIGenLib/Defloater  SystemSampleTime=-1  VariantActivationTime=update diagram  AllowFlexibleInterface=on  Latency=0  AutoFrameSizeCalculation=off
  Demux{,2..5} (5 alike) : Demux
  Demux1 : Demux  Outputs=5
  Display3 : Display
  Ethernet Setup Carla : dsmpblib/Data Inport  Priority=10000
      settings: SourceProductName=dSPACE Model Interface Package for Simulink (MIPS)
  Floater : VSIGenLib/Floater  SystemSampleTime=-1  VariantActivationTime=update diagram  AllowFlexibleInterface=on  Latency=0  AutoFrameSizeCalculation=off
  Floater1 : VSIGenLib/Floater  SystemSampleTime=-1  VariantActivationTime=update diagram  AllowFlexibleInterface=on  Latency=0  AutoFrameSizeCalculation=off
  Floater2 : VSIGenLib/Floater  SystemSampleTime=-1  VariantActivationTime=update diagram  AllowFlexibleInterface=on  Latency=0  AutoFrameSizeCalculation=off
  Mux : Mux  Inputs=21
  Mux1 : Mux  Inputs=3
  Receive [TCP Carla] : dsmpblib/Data Inport  Priority=10000
      settings: SourceProductName=dSPACE Model Interface Package for Simulink (MIPS)
  Scope1 : Scope
  Scope4 : Scope
  Selector1 : Selector  InputPortWidth=1024  IndexOptions=Index vector (dialog)  Indices=[8 7 6 5]  OutputSizes=1
  Selector2 : Selector  InputPortWidth=1024  IndexOptions=Index vector (dialog)  Indices=[12 11 10 9]  OutputSizes=1
  Selector4 : Selector  InputPortWidth=1024  IndexOptions=Index vector (dialog)  Indices=[4 3 2 1]  OutputSizes=1
  SpdAdjust : Gain  Gain=1.1414
  Status/Control_In [TCP Carla] : dsmpblib/Data Inport  Priority=10000
      settings: SourceProductName=dSPACE Model Interface Package for Simulink (MIPS)
  Status/Control_Out [TCP Carla] : dsmpblib/Data Outport  Priority=-10000
      settings: SourceProductName=dSPACE Model Interface Package for Simulink (MIPS)
  Terminator{1..5} (5 alike) : Terminator
  Transmit_In [TCP Carla] : dsmpblib/Data Inport  Priority=10000
      settings: SourceProductName=dSPACE Model Interface Package for Simulink (MIPS)
  Transmit_Out [TCP Carla] : dsmpblib/Data Outport  Priority=-10000
      settings: SourceProductName=dSPACE Model Interface Package for Simulink (MIPS)
  uint8 (unsigned 8) 4 : etargetslib/Byte Pack  datatypes={'uint8'}  byteAlign=1
  Output : Outport
  wires:
  Demux4/4 -> Mux/16
  Demux3/4 -> Mux/12
  Defloater1/1 -> Demux2/1
  Mux/1 -> Data Type Conversion2/1
  Demux4/2 -> Mux/14
  Demux3/1 -> Mux/9
  Demux/4 -> Mux/4
  Demux/1 -> Mux/1
  Demux2/4 -> Mux/8
  Demux1/3 -> Defloater2/1
  Defloater/1 -> Demux/1
  Defloater3/1 -> Demux4/1
  Demux3/3 -> Mux/11
  Demux1/2 -> Defloater1/1
  Demux2/2 -> Mux/6
  Constant2/1 -> uint8 (unsigned 8) 4/1
  Demux1/1 -> Defloater/1
  Defloater2/1 -> Demux3/1
  Demux1/4 -> Defloater3/1
  Demux3/2 -> Mux/10
  Demux/3 -> Mux/3
  Demux/2 -> Mux/2
  In1/1 -> Demux1/1
  Demux2/1 -> Mux/5
  Demux4/1 -> Mux/13
  Demux2/3 -> Mux/7
  Demux4/3 -> Mux/15
  Data Type Conversion2/1 -> Transmit_Out [TCP Carla]/1
  Transmit_In [TCP Carla]/2 -> Terminator2/1
  Transmit_In [TCP Carla]/1 -> Terminator1/1
  Receive [TCP Carla]/1 -> Selector4/1, Selector2/1, Selector1/1
  Selector4/1 -> Floater/1
  Floater/1 -> Display3/1, Mux1/1
  Receive [TCP Carla]/2 -> Terminator4/1
  Data Type Conversion3/1 -> Status/Control_Out [TCP Carla]/1
  In2/1 -> Data Type Conversion3/1
  Receive [TCP Carla]/4 -> Terminator5/1
  Receive [TCP Carla]/3 -> Terminator3/1
  Status/Control_In [TCP Carla]/1 -> Scope4/1
  Ethernet Setup Carla/1 -> Scope1/1
  Demux1/5 -> SpdAdjust/1
  Defloater4/1 -> Demux5/1
  Demux5/2 -> Mux/18
  Demux5/3 -> Mux/19
  Demux5/4 -> Mux/20
  uint8 (unsigned 8) 4/1 -> Mux/21
  Demux5/1 -> Mux/17
  SpdAdjust/1 -> Defloater4/1
  Selector1/1 -> Floater1/1
  Mux1/1 -> Data Type Conversion1/1
  Floater1/1 -> Mux1/2
  Selector2/1 -> Floater2/1
  Floater2/1 -> Mux1/3
  Data Type Conversion1/1 -> Output/1
